simulink model "buck_converter_CPM_closed_loop_simscape"  (R2016a)
settings: Solver=ode23tb  StartTime=0.0  StopTime=1e-3  MaxStep=1e-7  RelTol=1e-7
values from neighbouring files (symbols this model uses):
  C = 200e-6    (= 0.0002)    [buck_converter_CPM_closed_loop_simscape_parameters.m]
  C2 = 1/(2*pi*R2*fz)    [buck_converter_CPM_closed_loop_simscape_parameters.m]
  C3 = 1/(2*pi*R2*fp)    [buck_converter_CPM_closed_loop_simscape_parameters.m]
  Dmax = 0.9    [buck_converter_CPM_closed_loop_simscape_parameters.m]
  Dmin = 0    [buck_converter_CPM_closed_loop_simscape_parameters.m]
  fs = 1e6    (= 1000000)    [buck_converter_CPM_closed_loop_simscape_parameters.m]
  H = 0.6    [buck_converter_CPM_closed_loop_simscape_parameters.m]
  Imax = 5    [buck_converter_CPM_closed_loop_simscape_parameters.m]
  L = 1e-6    (= 1e-06)    [buck_converter_CPM_closed_loop_simscape_parameters.m]
  R1 = 1.2e3    (= 1200)    [buck_converter_CPM_closed_loop_simscape_parameters.m]
  R2 = Gcv0*R1    [buck_converter_CPM_closed_loop_simscape_parameters.m]
  Ra = (1/H-1)*Rb    (= 2000)    [buck_converter_CPM_closed_loop_simscape_parameters.m]
  Rb = R1/(1-H)    (= 3000)    [buck_converter_CPM_closed_loop_simscape_parameters.m]
  Resr = 0.8e-3    (= 0.0008)    [buck_converter_CPM_closed_loop_simscape_parameters.m]
  Rin = 10e6    (= 10000000)    [buck_converter_CPM_closed_loop_simscape_parameters.m]
  RL = 15e-3    (= 0.015)    [buck_converter_CPM_closed_loop_simscape_parameters.m]
  Rload = 3.7    [buck_converter_CPM_closed_loop_simscape_parameters.m]
  Rs = 0.3    [buck_converter_CPM_closed_loop_simscape_parameters.m]
  Va = Rs*ma*(1/fs)    (= 0.99)    [buck_converter_CPM_closed_loop_simscape_parameters.m]
  Vg = 5    [buck_converter_CPM_closed_loop_simscape_parameters.m]
  Vo = 3.3    [buck_converter_CPM_closed_loop_simscape_parameters.m]
undefined symbols (not defined in the file or in its folder): C3v
libraries: powerlib x52, simulink x1, simulink_extras x1
settings Model: Creator=Gorkem  LastModifiedBy=Gorkem
settings SolverCC: AlgebraicLoopSolver=LineSearch
settings DebuggingCC: MaxConsecutiveZCsMsg=none
settings GRTTargetCC: GeneratePreprocessorConditionals=Use local settings

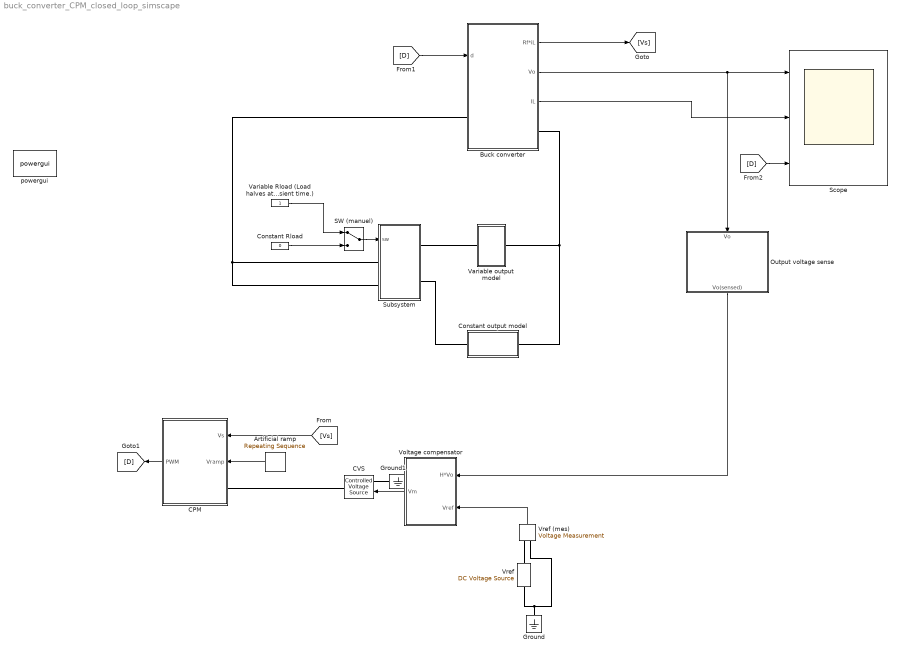
== system buck_converter_CPM_closed_loop_simscape ==
  Artificial ramp : simulink/Sources/Repeating Sequence  rep_seq_t=[0 0.999/fs 1/fs]  rep_seq_y=[0 Va 0]
  Buck converter : Subsystem
  CPM : Subsystem
  CVS : powerlib/Electrical Sources/Controlled Voltage Source  Initialize=off  Source_Type=AC  Amplitude=0  Phase=0  Frequency=0  Measurements=Voltage
  Constant Rload : Constant  Value=0
  Constant output model : Subsystem
  Ground : powerlib/Elements/Ground  LConnTagsString=a
  Ground1 : powerlib/Elements/Ground  LConnTagsString=a
  Output voltage sense : Subsystem
  SW (manuel) : ManualSwitch
  Scope : Scope  NumInputPorts=3
  Subsystem : Subsystem
  Variable Rload (Load halves at first and then increased to 1.5 times the rated value during transient time.) : Constant
  Variable output model : Subsystem
  Voltage compensator : Subsystem
  Vref : powerlib/Electrical Sources/DC Voltage Source  Amplitude=H*Vo  Measurements=None
  Vref (mes) : powerlib/Measurements/Voltage Measurement  PhasorSimulation=off  OutputType=Complex  PSBequivalent=0
  powergui : powerlib/powergui  Priority=1  SimulationMode=Continuous  SolverType=Tustin/Backward Euler (TBE)  SampleTime=1e-10  frequency=60  SPID=off  DisableSnubberDevices=off  DisableRonSwitches=off  DisableVfSwitches=off  SwTol=0  DisplayEquations=off  Interpol=off  ExternalGateDelay=off  methode=off  Ts=10  FunctionMessages=off  echomessages=off  HookPort=off  EnableUseOfTLC=off  x0status=blocks  frequencyindice=0  Pbase=100e6  ErrMax=1e-4  Iterations=50  UnitsV=kV  UnitsW=MW  buscounter=0  RestoreLinks=warning  ResistiveCurrentMeasurement=off  Frange=[0:2:500]  Ylog=off  Xlog=on  ShowGrid=off  save=off  variable=ZData  structure=0  ZoomFFT=off  StartTime=0.0  cycles=1  DisplayStyle=1  fundamental=60  FreqAxis=off  MaxFrequency=1000  frequencyindicesteady=1  RmsSteady=1  display=off
  wires:
  Buck converter/2(Vo) -> Scope/1, Output voltage sense/1(Vo)
  Buck converter/3(IL) -> Scope/2
  Buck converter/1(Rf*iL) -> [Vs]
  [Vs] -> CPM/1(Vs)
  Artificial ramp/1 -> CPM/2(Vramp)
  Output voltage sense/1(Vo(sensed)) -> Voltage compensator/1(H*Vo)
  Vref (mes)/1 -> Voltage compensator/2(Vref)
  Voltage compensator/1(Vm) -> CVS/1
  Variable Rload (Load halves at first and then increased to 1.5 times the rated value during transient time.)/1 -> SW (manuel)/1
  Constant Rload/1 -> SW (manuel)/2
  SW (manuel)/1 -> Subsystem/1(sw)
  CPM/1(PWM) -> [D]
  [D] -> Buck converter/1(d)
  [D] -> Scope/3
  connections:
  Vref (mes)/LConn1 -- Vref/RConn1
  Ground/LConn1 -- Vref (mes)/LConn2 -- Vref/LConn1
  Ground1/LConn1 -- CVS/LConn1
  CVS/RConn1 -- CPM/LConn1
  Variable output model/RConn1 -- Constant output model/LConn1 -- Buck converter/RConn1
  Subsystem/LConn1 -- Subsystem/LConn2 -- Buck converter/LConn1
  Variable output model/LConn1 -- Subsystem/RConn1
  Constant output model/RConn1 -- Subsystem/RConn2

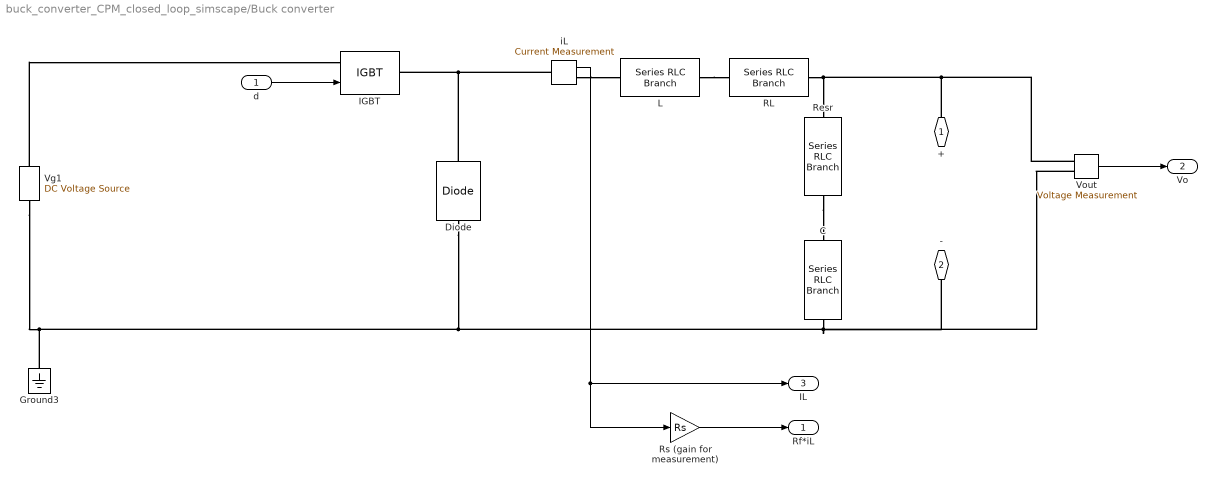
== system buck_converter_CPM_closed_loop_simscape/Buck converter ==
  d : Inport
  C : powerlib/Elements/Series RLC Branch  LConnTagsString=__new0  RConnTagsString=__new0  BranchType=C  Resistance=1  Inductance=L  SetiL0=off  InitialCurrent=0  Capacitance=C  Setx0=off  InitialVoltage=0  Measurements=None
  Diode : powerlib/Power Electronics/Diode  Ron=0.001  Lon=0  Vf=0.6  IC=0  UseSnubber=off  Rs=500  Cs=250e-9  Measurements=off
  Ground3 : powerlib/Elements/Ground  LConnTagsString=a
  IGBT : powerlib/Power Electronics/IGBT  Ron=0.001  Lon=0  Vf=0.5  Tf=1e-6  Tt=2e-6  IC=0  Rs=1e5  Cs=inf  Measurements=off
  L : powerlib/Elements/Series RLC Branch  LConnTagsString=__new0  RConnTagsString=__new0  BranchType=L  Resistance=1  Inductance=L  SetiL0=off  InitialCurrent=0  Capacitance=1e-6  Setx0=off  InitialVoltage=0  Measurements=None
  RL : powerlib/Elements/Series RLC Branch  LConnTagsString=__new0  RConnTagsString=__new0  BranchType=R  Resistance=RL  Inductance=L  SetiL0=off  InitialCurrent=0  Capacitance=C  Setx0=off  InitialVoltage=0  Measurements=None
  Resr : powerlib/Elements/Series RLC Branch  LConnTagsString=__new0  RConnTagsString=__new0  BranchType=R  Resistance=Resr  Inductance=L  SetiL0=off  InitialCurrent=0  Capacitance=C  Setx0=off  InitialVoltage=0  Measurements=None
  Rs (gain for measurement) : Gain  Gain=Rs
  Vg1 : powerlib/Electrical Sources/DC Voltage Source  Amplitude=Vg  Measurements=None
  Vout : powerlib/Measurements/Voltage Measurement  PhasorSimulation=off  OutputType=Complex  PSBequivalent=0
  iL : powerlib/Measurements/Current Measurement  PhasorSimulation=off  OutputType=Complex  PSBequivalent=0
  + : PMIOPort  Port=1  Side=Left
  - : PMIOPort  Port=2  Side=Right
  Rf*iL : Outport
  Vo : Outport  Port=2
  IL : Outport  Port=3
  wires:
  Rs (gain for measurement)/1 -> Rf*iL/1
  iL/1 -> IL/1, Rs (gain for measurement)/1
  Vout/1 -> Vo/1
  d/1 -> IGBT/1
  connections:
  Vg1/LConn1 -- Diode/LConn1 -- Vout/LConn2 -- -/RConn1 -- C/RConn1 -- Ground3/LConn1
  Diode/RConn1 -- iL/LConn1 -- IGBT/RConn1
  Vout/LConn1 -- RL/RConn1 -- Resr/LConn1 -- +/RConn1
  Vg1/RConn1 -- IGBT/LConn1
  L/RConn1 -- RL/LConn1
  iL/RConn1 -- L/LConn1
  Resr/RConn1 -- C/LConn1

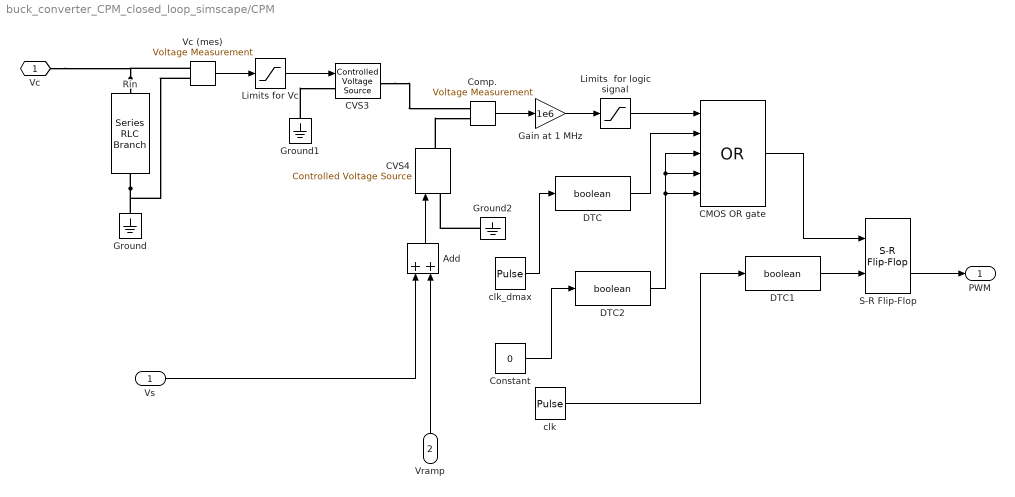
== system buck_converter_CPM_closed_loop_simscape/CPM ==
  Vs : Inport
  Vramp : Inport  Port=2
  Add : Sum
  CMOS OR gate : Logic  Operator=OR  Inputs=5  AllPortsSameDT=off  OutDataTypeStr=boolean
  CVS3 : powerlib/Electrical Sources/Controlled Voltage Source  Initialize=off  Source_Type=AC  Amplitude=0  Phase=0  Frequency=0  Measurements=Voltage
  CVS4 : powerlib/Electrical Sources/Controlled Voltage Source  Initialize=off  Source_Type=AC  Amplitude=0  Phase=0  Frequency=0  Measurements=Voltage
  Comp. : powerlib/Measurements/Voltage Measurement  PhasorSimulation=off  OutputType=Complex  PSBequivalent=0
  Constant : Constant  Value=0
  DTC : DataTypeConversion  OutDataTypeStr=boolean  SaturateOnIntegerOverflow=on  LockScale=on
  DTC1 : DataTypeConversion  OutDataTypeStr=boolean  SaturateOnIntegerOverflow=on  LockScale=on
  DTC2 : DataTypeConversion  OutDataTypeStr=boolean  SaturateOnIntegerOverflow=on  LockScale=on
  Gain at 1 MHz : Gain  Gain=1e6
  Ground : powerlib/Elements/Ground  LConnTagsString=a
  Ground1 : powerlib/Elements/Ground  LConnTagsString=a
  Ground2 : powerlib/Elements/Ground  LConnTagsString=a
  Limits for Vc : Saturate  UpperLimit=Imax*Rs  LowerLimit=-inf  ZeroCross=off
  "Limits  for logic signal " : Saturate  UpperLimit=1  LowerLimit=0
  Rin : powerlib/Elements/Series RLC Branch  LConnTagsString=__new0  RConnTagsString=__new0  BranchType=R  Resistance=Rin  Inductance=1e-3  SetiL0=off  InitialCurrent=0  Capacitance=1e-6  Setx0=off  InitialVoltage=0  Measurements=None
  S-R Flip-Flop : simulink_extras/Flip Flops/S-R Flip-Flop  initial_condition=0
  Vc (mes) : powerlib/Measurements/Voltage Measurement  PhasorSimulation=off  OutputType=Complex  PSBequivalent=0
  clk : DiscretePulseGenerator  PulseType=Time based  Amplitude=5  Period=1/fs  PulseWidth=(Dmin+1e-10)*100
  clk_dmax : DiscretePulseGenerator  PulseType=Time based  Amplitude=5  Period=1/fs  PulseWidth=(1-Dmax)*100  PhaseDelay=Dmax/fs
  Vc : PMIOPort  Port=1  Side=Left
  PWM : Outport
  wires:
  Vs/1 -> Add/1
  Add/1 -> CVS4/1
  Limits for Vc/1 -> CVS3/1
  Vramp/1 -> Add/2
  Vc (mes)/1 -> Limits for Vc/1
  Comp./1 -> Gain at 1 MHz/1
  Gain at 1 MHz/1 -> "Limits  for logic signal "/1
  S-R Flip-Flop/2 -> PWM/1
  CMOS OR gate/1 -> S-R Flip-Flop/1
  clk_dmax/1 -> DTC/1
  DTC/1 -> CMOS OR gate/2
  DTC1/1 -> S-R Flip-Flop/2
  clk/1 -> DTC1/1
  Constant/1 -> DTC2/1
  DTC2/1 -> CMOS OR gate/5, CMOS OR gate/4, CMOS OR gate/3
  "Limits  for logic signal "/1 -> CMOS OR gate/1
  connections:
  Rin/RConn1 -- Ground/LConn1 -- Vc (mes)/LConn2
  Rin/LConn1 -- Vc (mes)/LConn1 -- Vc/RConn1
  CVS4/RConn1 -- Comp./LConn1
  Ground2/LConn1 -- CVS4/LConn1
  Ground1/LConn1 -- CVS3/LConn1
  CVS3/RConn1 -- Comp./LConn2

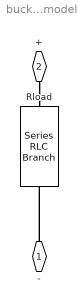
== system buck_converter_CPM_closed_loop_simscape/Constant output model ==
  Rload : powerlib/Elements/Series RLC Branch  LConnTagsString=__new0  RConnTagsString=__new0  BranchType=R  Resistance=Rload  Inductance=L  SetiL0=off  InitialCurrent=0  Capacitance=1e-6  Setx0=off  InitialVoltage=0  Measurements=None
  - : PMIOPort  Port=1  Side=Left
  + : PMIOPort  Port=2  Side=Right
  connections:
  -/RConn1 -- Rload/RConn1
  +/RConn1 -- Rload/LConn1

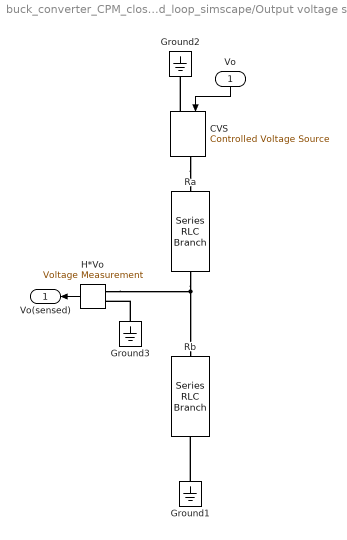
== system buck_converter_CPM_closed_loop_simscape/Output voltage sense ==
  Vo : Inport
  CVS : powerlib/Electrical Sources/Controlled Voltage Source  Initialize=on  Source_Type=AC  Amplitude=0  Phase=0  Frequency=0  Measurements=None
  Ground1 : powerlib/Elements/Ground  LConnTagsString=a
  Ground2 : powerlib/Elements/Ground  LConnTagsString=a
  Ground3 : powerlib/Elements/Ground  LConnTagsString=a
  H*Vo : powerlib/Measurements/Voltage Measurement  PhasorSimulation=off  OutputType=Complex  PSBequivalent=0
  Ra : powerlib/Elements/Series RLC Branch  LConnTagsString=__new0  RConnTagsString=__new0  BranchType=R  Resistance=Ra  Inductance=1e-3  SetiL0=off  InitialCurrent=0  Capacitance=C3  Setx0=off  InitialVoltage=0  Measurements=None
  Rb : powerlib/Elements/Series RLC Branch  LConnTagsString=__new0  RConnTagsString=__new0  BranchType=R  Resistance=Rb  Inductance=1e-3  SetiL0=off  InitialCurrent=0  Capacitance=C3  Setx0=off  InitialVoltage=0  Measurements=None
  Vo(sensed) : Outport
  wires:
  H*Vo/1 -> Vo(sensed)/1
  Vo/1 -> CVS/1
  connections:
  Ra/RConn1 -- Rb/LConn1 -- H*Vo/LConn1
  Ground1/LConn1 -- Rb/RConn1
  Ground3/LConn1 -- H*Vo/LConn2
  CVS/RConn1 -- Ra/LConn1
  CVS/LConn1 -- Ground2/LConn1

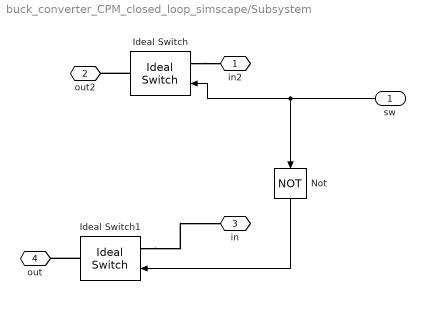
== system buck_converter_CPM_closed_loop_simscape/Subsystem ==
  sw : Inport
  Ideal Switch : powerlib/Power Electronics/Ideal Switch  Ron=1e-10  Lon=0  IC=0  Rs=1e5  Cs=inf  Measurements=off
  Ideal Switch1 : powerlib/Power Electronics/Ideal Switch  Ron=1e-10  Lon=0  IC=0  Rs=1e5  Cs=inf  Measurements=off
  Not : Logic  Operator=NOT  AllPortsSameDT=off  OutDataTypeStr=boolean
  in2 : PMIOPort  Port=1  Side=Right
  out2 : PMIOPort  Port=2  Side=Left
  in : PMIOPort  Port=3  Side=Right
  out : PMIOPort  Port=4  Side=Left
  wires:
  sw/1 -> Ideal Switch/1, Not/1
  Not/1 -> Ideal Switch1/1
  connections:
  Ideal Switch1/RConn1 -- out/RConn1
  Ideal Switch1/LConn1 -- in/RConn1
  Ideal Switch/LConn1 -- in2/RConn1
  Ideal Switch/RConn1 -- out2/RConn1

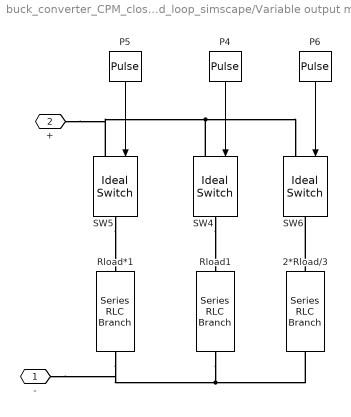
== system buck_converter_CPM_closed_loop_simscape/Variable output model ==
  2*Rload/3 : powerlib/Elements/Series RLC Branch  LConnTagsString=__new0  RConnTagsString=__new0  BranchType=R  Resistance=2*Rload/3  Inductance=L  SetiL0=off  InitialCurrent=0  Capacitance=1e-6  Setx0=off  InitialVoltage=0  Measurements=None
  P4 : DiscretePulseGenerator  PulseType=Time based  Period=1e-3  PulseWidth=60
  P5 : DiscretePulseGenerator  PulseType=Time based  Period=(0.12/0.2)*1e-3  PulseWidth=33  PhaseDelay=(0.04/0.2)*1e-3
  P6 : DiscretePulseGenerator  PulseType=Time based  Period=1e-3  PulseWidth=20  PhaseDelay=(0.12/0.2)*1e-3
  Rload*1 : powerlib/Elements/Series RLC Branch  LConnTagsString=__new0  RConnTagsString=__new0  BranchType=R  Resistance=Rload  Inductance=L  SetiL0=off  InitialCurrent=0  Capacitance=1e-6  Setx0=off  InitialVoltage=0  Measurements=None
  Rload1 : powerlib/Elements/Series RLC Branch  LConnTagsString=__new0  RConnTagsString=__new0  BranchType=R  Resistance=Rload  Inductance=L  SetiL0=off  InitialCurrent=0  Capacitance=1e-6  Setx0=off  InitialVoltage=0  Measurements=None
  SW4 : powerlib/Power Electronics/Ideal Switch  Ron=1e-10  Lon=0  IC=0  Rs=1e5  Cs=inf  Measurements=off
  SW5 : powerlib/Power Electronics/Ideal Switch  Ron=1e-10  Lon=0  IC=0  Rs=1e5  Cs=inf  Measurements=off
  SW6 : powerlib/Power Electronics/Ideal Switch  Ron=1e-10  Lon=0  IC=0  Rs=1e5  Cs=inf  Measurements=off
  - : PMIOPort  Port=1  Side=Right
  + : PMIOPort  Port=2  Side=Left
  wires:
  P5/1 -> SW5/1
  P6/1 -> SW6/1
  P4/1 -> SW4/1
  connections:
  SW4/RConn1 -- Rload1/LConn1
  SW5/RConn1 -- Rload*1/LConn1
  2*Rload/3/LConn1 -- SW6/RConn1
  SW4/LConn1 -- SW5/LConn1 -- +/RConn1 -- SW6/LConn1
  Rload1/RConn1 -- 2*Rload/3/RConn1 -- Rload*1/RConn1 -- -/RConn1

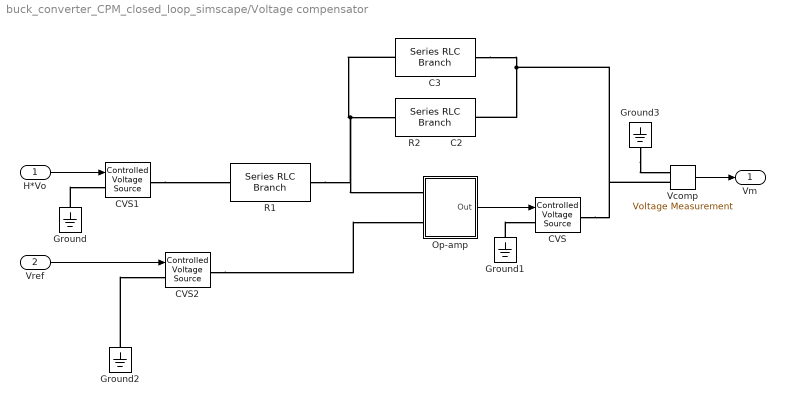
== system buck_converter_CPM_closed_loop_simscape/Voltage compensator ==
  H*Vo : Inport
  Vref : Inport  Port=2
  C3 : powerlib/Elements/Series RLC Branch  LConnTagsString=__new0  RConnTagsString=__new0  BranchType=C  Resistance=1  Inductance=1e-3  SetiL0=off  InitialCurrent=0  Capacitance=C3  Setx0=off  InitialVoltage=0  Measurements=None
  CVS : powerlib/Electrical Sources/Controlled Voltage Source  Initialize=off  Source_Type=AC  Amplitude=0  Phase=0  Frequency=0  Measurements=Voltage
  CVS1 : powerlib/Electrical Sources/Controlled Voltage Source  Initialize=off  Source_Type=DC  Amplitude=0  Phase=0  Frequency=0  Measurements=Voltage
  CVS2 : powerlib/Electrical Sources/Controlled Voltage Source  Initialize=off  Source_Type=DC  Amplitude=0  Phase=0  Frequency=0  Measurements=Voltage
  Ground{,1..3} (4 alike) : powerlib/Elements/Ground  LConnTagsString=a
  Op-amp : Subsystem
  R1 : powerlib/Elements/Series RLC Branch  LConnTagsString=__new0  RConnTagsString=__new0  BranchType=R  Resistance=R1  Inductance=1e-3  SetiL0=off  InitialCurrent=0  Capacitance=C3v  Setx0=off  InitialVoltage=0  Measurements=None
  R2          C2 : powerlib/Elements/Series RLC Branch  LConnTagsString=__new0  RConnTagsString=__new0  BranchType=RC  Resistance=R2  Inductance=1e-3  SetiL0=off  InitialCurrent=0  Capacitance=C2  Setx0=off  InitialVoltage=0  Measurements=None
  Vcomp : powerlib/Measurements/Voltage Measurement  PhasorSimulation=off  OutputType=Complex  PSBequivalent=0
  Vm : Outport
  wires:
  Vref/1 -> CVS2/1
  H*Vo/1 -> CVS1/1
  Vcomp/1 -> Vm/1
  Op-amp/1(Out) -> CVS/1
  connections:
  Ground3/LConn1 -- Vcomp/LConn2
  Ground/LConn1 -- CVS1/LConn1
  Ground1/LConn1 -- CVS/LConn1
  Ground2/LConn1 -- CVS2/LConn1
  C3/LConn1 -- Op-amp/LConn1 -- R1/RConn1 -- R2          C2/LConn1
  C3/RConn1 -- Vcomp/LConn1 -- CVS/RConn1 -- R2          C2/RConn1
  CVS2/RConn1 -- Op-amp/LConn2
  CVS1/RConn1 -- R1/LConn1

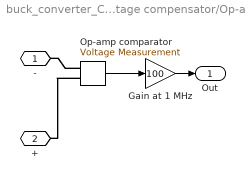
== system buck_converter_CPM_closed_loop_simscape/Voltage compensator/Op-amp ==
  Gain at 1 MHz : Gain  Gain=100
  "Op-amp comparator " : powerlib/Measurements/Voltage Measurement  PhasorSimulation=off  OutputType=Complex  PSBequivalent=0
  - : PMIOPort  Port=1  Side=Left
  + : PMIOPort  Port=2  Side=Left
  Out : Outport
  wires:
  Gain at 1 MHz/1 -> Out/1
  "Op-amp comparator "/1 -> Gain at 1 MHz/1
  connections:
  "Op-amp comparator "/LConn1 -- +/RConn1
  "Op-amp comparator "/LConn2 -- -/RConn1
